simulink model "FullBridgeACDCconverter"  (R2021a)
settings: Solver=VariableStepAuto  StartTime=0.0  StopTime=10.0  RelTol=1e-3
libraries: spsDiodeLib x8, spsSeriesRLCBranchLib x4, spsCurrentMeasurementLib x2, spsMosfetLib x2, spsParallelRLCLoadLib x2, eePowerMeasurement x2, spsRMSLib x2, spsVoltageMeasurementLib x2, spsACVoltageSourceLib x1, spsBreakerLib x1, simulink x1, pid_lib x1
settings Model: Creator=Administrator  LastModifiedBy=Halil
settings SolverCC: ZeroCrossAlgorithm=Adaptive  AlgebraicLoopSolver=TrustRegion
settings DebuggingCC: IgnoredZcDiagnostic=none  SFMachineParentedDataDiag=warning
settings SFSimCC: CustomCodeUndefinedFunction=UseInterfaceOnly

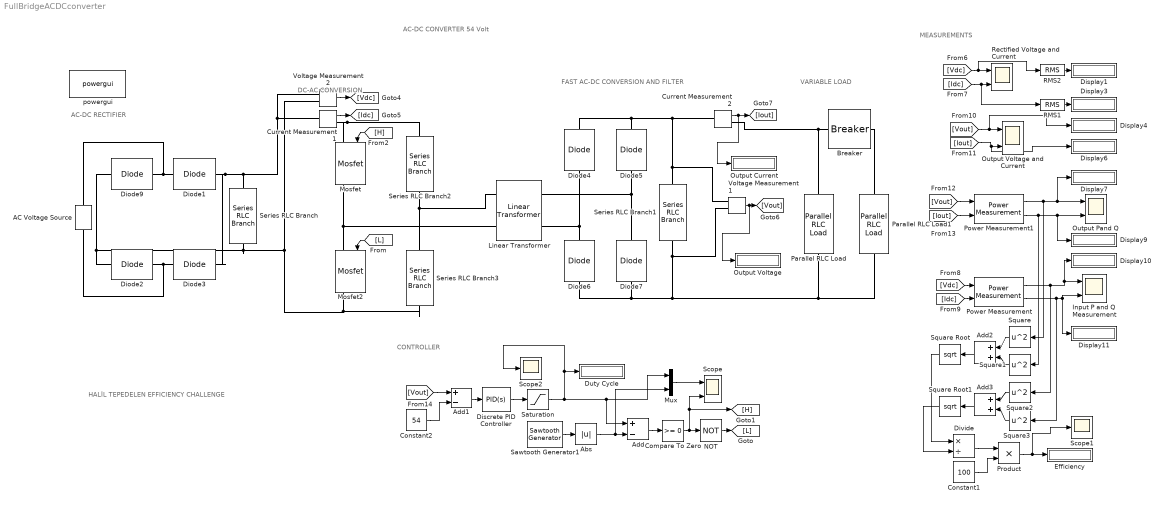
== system FullBridgeACDCconverter ==
  note: AC-DC CONVERTER 54 Volt
  note: HALİL TEPEDELEN
      | EFFICIENCY CHALLENGE
  note: CONTROLLER
  note: MEASUREMENTS
  note: DC-AC CONVERSION
  note: AC-DC RECTIFIER
  note: FAST AC-DC CONVERSION AND
      | FILTER
  note: VARIABLE LOAD
  AC Voltage Source : spsACVoltageSourceLib/AC Voltage Source  Amplitude=311  Phase=0  Frequency=50  SampleTime=0  Measurements=None  BusType=swing  Pref=10e3  Qref=0  Qmin=-inf  Qmax=+inf
  Abs : Abs
  Add : Sum  Inputs=+-
  Add1 : Sum  Inputs=+-
  Add2 : Sum
  Add3 : Sum
  Breaker : spsBreakerLib/Breaker  InitialState=1  SwitchingTimes=[0]  External=off  BreakerResistance=0.000000001  SnubberResistance=1e6  SnubberCapacitance=inf  Measurements=None  MoreParameters=on  NoBreakLoop=off
      settings: SourceProductBaseCode=PS
  Compare To Zero : simulink/Logic and Bit Operations/Compare To Zero  relop=>=  OutDataTypeStr=boolean
  Constant1 : Constant  Value=100
  Constant2 : Constant  Value=54
  Current Measurement1 : spsCurrentMeasurementLib/Current Measurement  PhasorSimulation=off  OutputType=Complex  PSBequivalent=0
  Current Measurement2 : spsCurrentMeasurementLib/Current Measurement  PhasorSimulation=off  OutputType=Complex  PSBequivalent=0
  Diode{1..7,9} (8 alike) : spsDiodeLib/Diode  Ron=0.001  Lon=0  Vf=0.8  IC=0  UseSnubber=0  Rs=500  Cs=250e-9  Measurements=off
  Discrete PID Controller : pid_lib/PID Controller  Controller=PID  Form=Parallel  TimeDomain=Continuous-time  UseExternalTs=off  SampleTime=-1  IntegratorMethod=Forward Euler  FilterMethod=Forward Euler  ControllerParametersSource=internal  P=1  I=1  D=0  UseFilter=on  N=100000  TunerSelectOption=Transfer Function Based (PID Tuner App)  InitialConditionSource=internal  InitialConditionForIntegrator=0  InitialConditionForFilter=0  DifferentiatorICPrevScaledInput=0  ExternalReset=none  TrackingMode=off  Kt=1  LimitOutput=on  SatLimitsSource=internal  UpperSaturationLimit=inf  LowerSaturationLimit=0.25  LinearizeAsGain=off  AntiWindupMode=none  Kb=1  POutMin=[]  POutMax=[]  IOutMin=[]  IOutMax=[]  DOutMin=[]  DOutMax=[]  NOutMin=[]  NOutMax=[]  SumOutMin=[]  SumOutMax=[]  SaturationOutMin=[]  SaturationOutMax=[]  PParamMin=[]  PParamMax=[]  IParamMin=[]  IParamMax=[]  DParamMin=[]  DParamMax=[]  NParamMin=[]  NParamMax=[]  KbParamMin=[]  KbParamMax=[]  KtParamMin=[]  KtParamMax=[]  KbOutMin=[]  KbOutMax=[]  KtOutMin=[]  KtOutMax=[]  IntegratorOutMin=[]  IntegratorOutMax=[]  FilterOutMin=[]  FilterOutMax=[]  SumI1OutMin=[]  SumI1OutMax=[]  SumI2OutMin=[]  SumI2OutMax=[]  SumI3OutMin=[]  SumI3OutMax=[]  SumI4OutMin=[]  SumI4OutMax=[]  SumDOutMin=[]  SumDOutMax=[]  DifferentiatorOutMin=[]  DifferentiatorOutMax=[]  FilterDiffOutCoefMin=[]  FilterDiffOutCoefMax=[]  ReciprocalOutMin=[]  ReciprocalOutMax=[]  SumDenOutMin=[]  SumDenOutMax=[]  SumNumOutMin=[]  SumNumOutMax=[]  DivideOutMin=[]  DivideOutMax=[]  UdiffTsProdOutMin=[]  UdiffTsProdOutMax=[]  NTsProdOutMin=[]  NTsProdOutMax=[]  UintegralTsProdOutMin=[]  UintegralTsProdOutMax=[]  UngainTsProdOutMin=[]  UngainTsProdOutMax=[]  IntegratorContinuousStateAttributes=''  IntegratorStateMustResolveToSignalObject=off  IntegratorRTWStateStorageClass=Auto  FilterContinuousStateAttributes=''  FilterStateMustResolveToSignalObject=off  FilterRTWStateStorageClass=Auto  ParallelPVariant=InternalParameters  IdealPVariant=Disabled  IVariant=InternalParameters  DVariant=InternalParameters  IntegratorVariant=Continuous  SatVariant=Enabled  AWVariant=Passthrough  PCopyVariant=Disabled  TRVariant=Disabled  FdbkBlocksVariant=Forward  IdealPFdbkVariant=Disabled  SatFdbkVariant=Disabled  DerivativeFilterVariant=ContFilter  NVariant=InternalParameters  NCopyVariant=Disabled  FilterICVariant=InternalICsFilter  IntegratorICVariant=InternalICs  ExternalResetVariant=Disabled  TRSumVariant=Passthrough  SumFdbkVariant=Disabled  SumVariant=Sum_PID  TsampFilterVariant=InternalTs  TsampNgainVariant=Passthrough  TsampIntegralVariant=Passthrough  ExternalSaturationOutDataTypeStr=Inherit: Same as second input
  Display{1,3..4,6..7,9..11} (8 alike) : Display
  Divide : Product  Inputs=*/  RndMeth=Zero  SaturateOnIntegerOverflow=on
  Duty Cycle : Display
  Efficiency : Display
  Input P and Q Measurement : Scope  NumInputPorts=2
  Linear Transformer : spsLinearTransformerLib/Linear Transformer  UNITS=pu  NominalPower=[ 2000 1e3 ]  winding1="[70  0.002  0.08 ]"  winding2="[ 60 0.002  0.08 ]"  ThreeWindings=off  winding3=[ 315e3 0.002 0.08 ]  RmLm=[ 500 500 ]  Measurements=None  DataType=off
  Mosfet : spsMosfetLib/Mosfet  Ron=0.1  Lon=0  Rd=0.01  Vfd=0  IC=0  Rs=1e5  Cs=inf  Measurements=on
  Mosfet2 : spsMosfetLib/Mosfet  Ron=0.1  Lon=0  Rd=0.01  Vfd=0  IC=0  Rs=1e5  Cs=inf  Measurements=on
  Mux : Mux  Inputs=2
  NOT : Logic  Operator=NOT  IconShape=distinctive  AllPortsSameDT=off  OutDataTypeStr=boolean
  Output Current : Display
  Output Pand Q : Scope  NumInputPorts=2
  Output Voltage : Display
  Output Voltage and Current : Scope  NumInputPorts=2
  Parallel RLC Load : spsParallelRLCLoadLib/Parallel RLC Load  LConnTagsString=a  RConnTagsString=__new0  NominalVoltage=24  NominalFrequency=1000  ActivePower=1000  InductivePower=0  CapacitivePower=0  Setx0=off  InitialVoltage=0  SetiL0=off  InitialCurrent=0  Measurements=None  LoadType=constant Z
      settings: AttributesFormatString=\n  SourceProductBaseCode=PS
  Parallel RLC Load1 : spsParallelRLCLoadLib/Parallel RLC Load  LConnTagsString=a  RConnTagsString=__new0  NominalVoltage=24  NominalFrequency=1000  ActivePower=1000  InductivePower=0  CapacitivePower=0  Setx0=off  InitialVoltage=0  SetiL0=off  InitialCurrent=0  Measurements=None  LoadType=constant Z
      settings: AttributesFormatString=\n  SourceProductBaseCode=PS
  Power Measurement : eePowerMeasurement/Power Measurement  LabelModeActiveChoice=Continuous  F=60  K=[0 1 2 3]  Ts=0
      settings: SourceProductBaseCode=PS
  Power Measurement1 : eePowerMeasurement/Power Measurement  LabelModeActiveChoice=Continuous  F=60  K=[0 1 2 3]  Ts=0
      settings: SourceProductBaseCode=PS
  Product : Product
  RMS1 : spsRMSLib/RMS  TrueRMS=on  Freq=50  RMSInit=0  Ts=0
  RMS2 : spsRMSLib/RMS  TrueRMS=on  Freq=50  RMSInit=0  Ts=0
  Rectified Voltage and Current : Scope  NumInputPorts=2
  Saturation : Saturate  UpperLimit=0.9  LowerLimit=0  LinearizeAsGain=off
  Sawtooth Generator1 : spsSawtoothGeneratorLib/Sawtooth Generator  Freq=1e3  Phase=0  Ts=0
  Scope : Scope  NumInputPorts=2
  Scope1 : Scope
  Scope2 : Scope
  Series RLC Branch : spsSeriesRLCBranchLib/Series RLC Branch  LConnTagsString=__new0  RConnTagsString=__new0  BranchType=C  Resistance=1  Inductance=1e-3  SetiL0=off  InitialCurrent=0  Capacitance=30000e-6  Setx0=off  InitialVoltage=0  Measurements=None
  Series RLC Branch1 : spsSeriesRLCBranchLib/Series RLC Branch  LConnTagsString=__new0  RConnTagsString=__new0  BranchType=C  Resistance=1  Inductance=1e-3  SetiL0=off  InitialCurrent=0  Capacitance=90000e-6  Setx0=off  InitialVoltage=20  Measurements=None
  Series RLC Branch2 : spsSeriesRLCBranchLib/Series RLC Branch  LConnTagsString=__new0  RConnTagsString=__new0  BranchType=C  Resistance=1  Inductance=1e-3  SetiL0=off  InitialCurrent=0  Capacitance=30000e-6  Setx0=off  InitialVoltage=0  Measurements=None
  Series RLC Branch3 : spsSeriesRLCBranchLib/Series RLC Branch  LConnTagsString=__new0  RConnTagsString=__new0  BranchType=C  Resistance=1  Inductance=1e-3  SetiL0=off  InitialCurrent=0  Capacitance=30000e-6  Setx0=off  InitialVoltage=0  Measurements=None
  Square{,1..3} (4 alike) : Math  Operator=square  SignedPower=on  SaturateOnIntegerOverflow=on
  Square Root : Sqrt  SaturateOnIntegerOverflow=on
  Square Root1 : Sqrt  SaturateOnIntegerOverflow=on
  Voltage Measurement1 : spsVoltageMeasurementLib/Voltage Measurement  PhasorSimulation=off  OutputType=Complex  PSBequivalent=0
  Voltage Measurement2 : spsVoltageMeasurementLib/Voltage Measurement  PhasorSimulation=off  OutputType=Complex  PSBequivalent=0
  powergui : spspowerguiLib/powergui  Priority=1  SimulationMode=Continuous  SampleTime=50e-6  frequency=60  Iterations=50  frequencyindice=50  Pbase=100e6  ErrMax=1e-4  UnitsV=kV  UnitsW=MW  buscounter=0  FunctionMessages=off  echomessages=off  EnableUseOfTLC=off  CurrentSourceSwitches=off  DisableSnubberDevices=off  DisableRonSwitches=off  DisableVfSwitches=off  DisplayEquations=off  AutomaticDiscreteSolvers=off  SolverType=Tustin/Backward Euler (TBE)  Interpol=off  ExternalGateDelay=off  methode=off  Ts=100  x0status=blocks  SPID=on  SwTol=0  HookPort=off  NonlinearTolerance=0  nMaxIteration=15  ContinueOnMaxIteration=off  RestoreLinks=warning  ResistiveCurrentMeasurement=off  Frange=[0:2:500]  Ylog=off  Xlog=on  ShowGrid=off  save=off  variable=ZData  structure=0  ZoomFFT=off  StartTime=0.0  cycles=1  DisplayStyle=1  fundamental=60  FreqAxis=off  MaxFrequency=1000  frequencyindicesteady=1  RmsSteady=1  display=off
  wires:
  Add/1 -> Compare To Zero/1
  Mux/1 -> Scope/1
  Sawtooth Generator1/1 -> Abs/1
  Abs/1 -> Mux/2, Add/2
  Compare To Zero/1 -> NOT/1, Scope/2, [H]
  NOT/1 -> [L]
  [L] -> Mosfet2/1
  [H] -> Mosfet/1
  Power Measurement/1 -> Square2/1, Display10/1, Input P and Q Measurement/1
  Power Measurement/2 -> Square3/1, Display11/1, Input P and Q Measurement/2
  Voltage Measurement2/1 -> [Vdc]
  Current Measurement1/1 -> [Idc]
  [Vdc] -> RMS2/1, Rectified Voltage and Current/1
  [Idc] -> RMS1/1, Rectified Voltage and Current/2
  [Vdc] -> Power Measurement/1
  [Idc] -> Power Measurement/2
  [Vout] -> Display4/1, Output Voltage and Current/1
  [Iout] -> Display6/1, Output Voltage and Current/2
  [Vout] -> Power Measurement1/1
  [Iout] -> Power Measurement1/2
  Power Measurement1/1 -> Display7/1, Output Pand Q/1, Square/1
  Power Measurement1/2 -> Display9/1, Output Pand Q/2, Square1/1
  RMS2/1 -> Display1/1
  RMS1/1 -> Display3/1
  Voltage Measurement1/1 -> Output Voltage/1, [Vout]
  Current Measurement2/1 -> Output Current/1, [Iout]
  Add1/1 -> Discrete PID Controller/1
  Square/1 -> Add2/1
  Square1/1 -> Add2/2
  Square2/1 -> Add3/1
  Square3/1 -> Add3/2
  Add2/1 -> Square Root/1
  Add3/1 -> Square Root1/1
  Square Root1/1 -> Divide/2
  Square Root/1 -> Divide/1
  Divide/1 -> Product/1
  Constant1/1 -> Product/2
  Product/1 -> Scope1/1, Efficiency/1
  Discrete PID Controller/1 -> Saturation/1
  Saturation/1 -> Add/1, Mux/1, Scope2/1, Duty Cycle/1
  [Vout] -> Add1/1
  Constant2/1 -> Add1/2
  connections:
  AC Voltage Source/LConn1 -- Diode3/LConn1 -- Diode2/RConn1
  Series RLC Branch3/RConn1 -- Mosfet2/RConn1 -- Voltage Measurement2/LConn2 -- Series RLC Branch/RConn1 -- Diode2/LConn1 -- Diode9/LConn1
  Voltage Measurement2/LConn1 -- Current Measurement1/LConn1 -- Series RLC Branch/LConn1 -- Diode3/RConn1 -- Diode1/RConn1
  Mosfet2/LConn1 -- Linear Transformer/LConn2 -- Mosfet/RConn1
  Diode6/LConn1 -- Diode7/LConn1 -- Parallel RLC Load1/RConn1 -- Parallel RLC Load/RConn1 -- Voltage Measurement1/LConn2 -- Series RLC Branch1/RConn1
  Current Measurement1/RConn1 -- Mosfet/LConn1 -- Series RLC Branch2/LConn1
  Current Measurement2/RConn1 -- Parallel RLC Load/LConn1 -- Breaker/LConn1
  Diode4/RConn1 -- Current Measurement2/LConn1 -- Voltage Measurement1/LConn1 -- Series RLC Branch1/LConn1 -- Diode5/RConn1
  Diode1/LConn1 -- AC Voltage Source/RConn1 -- Diode9/RConn1
  Diode6/RConn1 -- Diode4/LConn1 -- Linear Transformer/RConn2
  Diode7/RConn1 -- Linear Transformer/RConn1 -- Diode5/LConn1
  Parallel RLC Load1/LConn1 -- Breaker/RConn1
  Series RLC Branch3/LConn1 -- Series RLC Branch2/RConn1 -- Linear Transformer/LConn1
